simulink model "lab3_1"  (R2023b)
settings: Solver=VariableStepAuto  StartTime=0.0  StopTime=2  MaxStep=0.1  MinStep=0.004  RelTol=1e-3
libraries: simulink x1
settings Model: Creator=user  LastModifiedBy=Admin
settings SolverCC: InitialStep=0.004

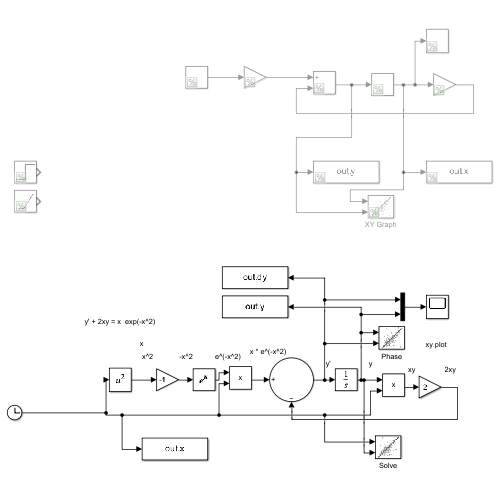
[thumbnail: Simulink's stored preview of the top-level diagram]
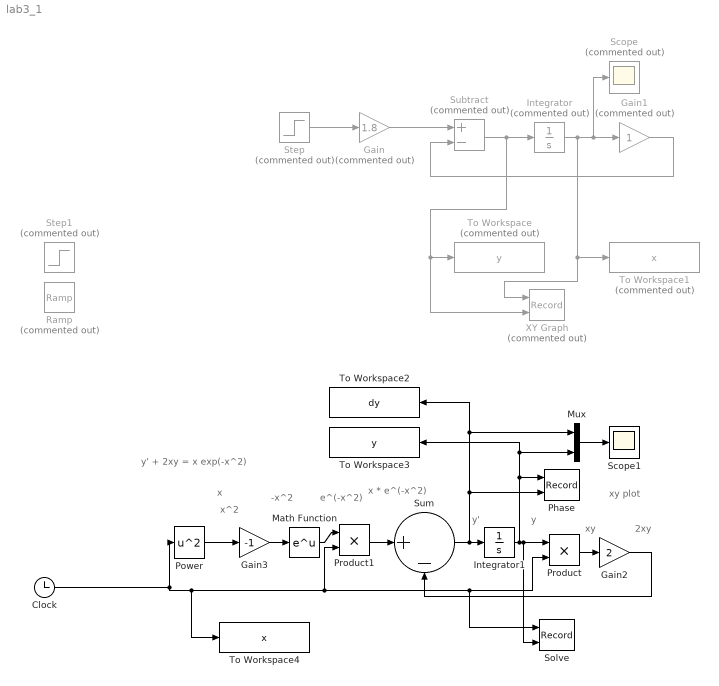
== system lab3_1 ==
  note: xy plot
  note: x * e^(-x^2)
  note: e^(-x^2)
  note: -x^2
  note: x^2
  note: 2xy
  note: xy
  note: y
  note: x
  note: y'
  note: y' + 2xy = x exp(-x^2)
  Clock : Clock
  Gain : Gain  Commented=on  Gain=1.8
  Gain1 : Gain  Commented=on
  Gain2 : Gain  Gain=2
  Gain3 : Gain  Gain=-1
  Integrator : Integrator  Commented=on
  Integrator1 : Integrator  InitialCondition=2
  Math Function : Math
  Mux : Mux  Inputs=2
  Phase : Record  FileSettingsInternal="{\"entries\":[{\"content\":{\"excelSettings\":{\"content\":{},\"type\":\"Streamout.ExcelSettings\"}},\"type\":\"Streamout.FileSettingStorage\",\"uuid\":\"\"}],\"packageUris\":[\"http:\\/\\/schema.mathworks.com\\/mf0\\/streamout_blocks\\/R2020a\"],\"version\":\"1.0\"}"  Layout=[1 1]  SignalsInternal="{\"entries\":[{\"content\":{\"signals\":[{\"content\":{\"blockPath\":[],\"dimensions\":[1],\"domain\":\"\",\"lineColor\":\"#b746ff\",\"port\":1,\"sid\":[\"\"],\"signalID\":526,\"signalName\":\"Integrator1\"},\"type\":\"RecordBlkView.Signal\",\"uuid\":\"\"},{\"content\":{\"blockPath\":[],\"dimensions\":[1],\"domain\":\"\",\"lineColor\":\"#64d413\",\"port\":2,\"sid\":[\"\"],\"signalID\":530,\"signalName\":\"Sum\"},\"type\":\"RecordBlkView.Signal\",\"uuid\":\"\"}]},\"type\":\"RecordBlkView.InputSignals\",\"uuid\":\"\"}],\"packageUris\":[\"http:\\/\\/schema.mathworks.com\\/mf0\\/streamout_blocks\\/R2020a\"],\"version\":\"1.0\"}"  VisualizationBindings="{\"xyplotplugin\":{\"info\":[{\"series\":[],\"subplotID\":1}]}}"  CompatibilityTag=XY
  Power : Math  Operator=square
  Product : Product
  Product1 : Product
  Ramp : simulink/Sources/Ramp  Commented=on  slope=0.004  start=0  InitialOutput=-2
  Scope : Scope  Commented=on
  Scope1 : Scope
  Solve : Record  FileSettingsInternal="{\"entries\":[{\"content\":{\"excelSettings\":{\"content\":{},\"type\":\"Streamout.ExcelSettings\"}},\"type\":\"Streamout.FileSettingStorage\",\"uuid\":\"\"}],\"packageUris\":[\"http:\\/\\/schema.mathworks.com\\/mf0\\/streamout_blocks\\/R2020a\"],\"version\":\"1.0\"}"  Layout=[1 1]  SignalsInternal="{\"entries\":[{\"content\":{\"signals\":[{\"content\":{\"blockPath\":[],\"dimensions\":[1],\"domain\":\"\",\"lineColor\":\"#a2142f\",\"plots\":[1],\"port\":1,\"sid\":[\"\"],\"signalID\":534,\"signalName\":\"Clock\"},\"type\":\"RecordBlkView.Signal\",\"uuid\":\"\"},{\"content\":{\"blockPath\":[],\"dimensions\":[1],\"domain\":\"\",\"lineColor\":\"#139fff\",\"plots\":[1],\"port\":2,\"sid\":[\"\"],\"signalID\":538,\"signalName\":\"Integrator1\"},\"type\":\"RecordBlkView.Signal\",\"uuid\":\"\"}]},\"type\":\"RecordBlkView.InputSignals\",\"uuid\":\"\"}],\"packageUris\":[\"http:\\/\\/schema.mathworks.com\\/mf0\\/streamout_blocks\\/R2020a\"],\"version\":\"1.0\"}"  VisualizationBindings="{\"xyplotplugin\":{\"info\":[{\"series\":[{\"bindingParametersList\":[{\"parameter\":\"X-Axis\",\"signalID\":534,\"signalName\":\"Clock\"},{\"parameter\":\"Y-Axis\",\"signalID\":538,\"signalName\":\"Integrator1\"}],\"seriesID\":20755}],\"subplotID\":1}]}}"  CompatibilityTag=XY
  Step : Step  Commented=on  SampleTime=0
  Step1 : Step  Commented=on  Time=0.004  Before=-2  After=2  SampleTime=0
  Subtract : Sum  Commented=on  Inputs=+-
  Sum : Sum  Inputs=|+-
  To Workspace : ToWorkspace  Commented=on  VariableName=y  SampleTime=-1
  To Workspace1 : ToWorkspace  Commented=on  VariableName=x  SampleTime=-1
  To Workspace2 : ToWorkspace  VariableName=dy  SampleTime=-1
  To Workspace3 : ToWorkspace  VariableName=y  SampleTime=-1
  To Workspace4 : ToWorkspace  VariableName=x  SampleTime=-1
  XY Graph : Record  Commented=on  FileSettingsInternal="{\"entries\":[{\"content\":{\"excelSettings\":{\"content\":{},\"type\":\"Streamout.ExcelSettings\"}},\"type\":\"Streamout.FileSettingStorage\",\"uuid\":\"\"}],\"packageUris\":[\"http:\\/\\/schema.mathworks.com\\/mf0\\/streamout_blocks\\/R2020a\"],\"version\":\"1.0\"}"  Layout=[1 1]  SignalsInternal="{\"entries\":[{\"content\":{},\"type\":\"RecordBlkView.InputSignals\",\"uuid\":\"\"}],\"packageUris\":[\"http:\\/\\/schema.mathworks.com\\/mf0\\/streamout_blocks\\/R2020a\"],\"version\":\"1.0\"}"  VisualizationBindings="{\"xyplotplugin\":{\"info\":[{\"series\":[],\"subplotID\":1}]}}"  CompatibilityTag=XY
  wires:
  Step/1 -> Gain/1
  Gain/1 -> Subtract/1
  Subtract/1 -> XY Graph/2, To Workspace/1, Integrator/1
  Integrator/1 -> XY Graph/1, To Workspace1/1, Scope/1, Gain1/1
  Gain1/1 -> Subtract/2
  Sum/1 -> To Workspace2/1, Mux/1, Phase/2, Integrator1/1
  Clock/1 -> To Workspace4/1, Product1/2, Solve/1, Product/2, Power/1
  Power/1 -> Gain3/1
  Integrator1/1 -> To Workspace3/1, Mux/2, Phase/1, Solve/2, Product/1
  Product/1 -> Gain2/1
  Gain2/1 -> Sum/2
  Gain3/1 -> Math Function/1
  Math Function/1 -> Product1/1
  Product1/1 -> Sum/1
  Mux/1 -> Scope1/1
